simulink model "simulacao"  (R2020b)
settings: Solver=VariableStepAuto  StartTime=0.0  StopTime=10.0  RelTol=1e-3
values from neighbouring files (symbols this model uses):
  i = 1    [teste.m]    (also in teste2.m)
  ki0 = 0.1    [teste.m]    (also in teste2.m = 0.2)
  kp0 = 0.1    [teste.m]    (also in teste2.m = 0.5)
  T = 0.01    [teste.m]    (also in teste2.m)
libraries: simulink x1
settings Model: Creator=luanh  LastModifiedBy=luanaraujo
settings DebuggingCC: AlgebraicLoopMsg=none

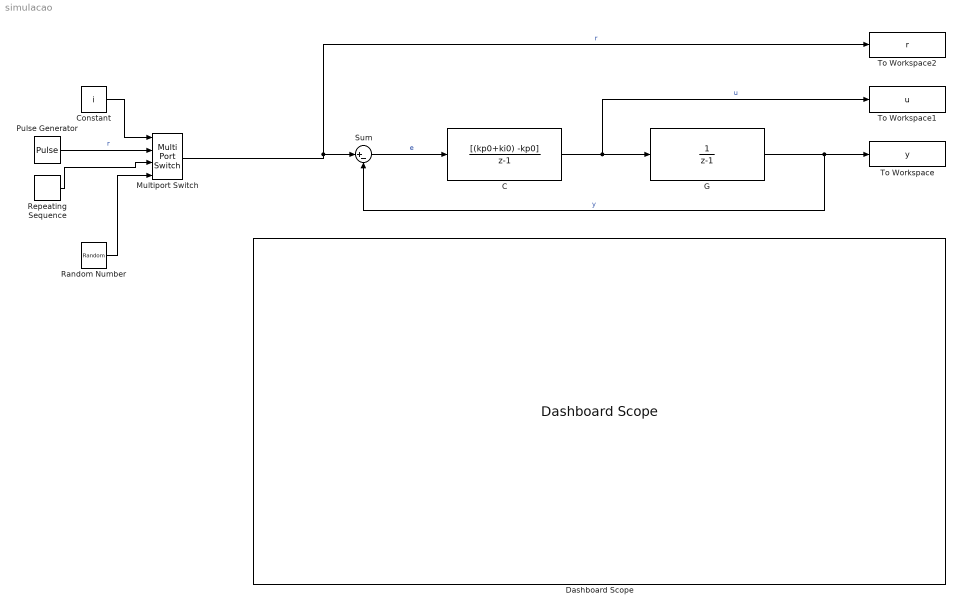
== system simulacao ==
  C : DiscreteTransferFcn  Numerator=[(kp0+ki0) -kp0]  Denominator=[1 -1]  SampleTime=T
  Constant : Constant  Value=i
  Dashboard Scope : DashboardScope
  G : DiscreteTransferFcn  Denominator=[1 -1]  SampleTime=T
  Multiport Switch : MultiPortSwitch
  Pulse Generator : DiscretePulseGenerator  PulseType=Time based  PulseWidth=50
  Random Number : RandomNumber  SampleTime=1
  Repeating Sequence : simulink/Sources/Repeating Sequence  rep_seq_t=[0 2]  rep_seq_y=[0 2]
  Sum : Sum  Inputs=|+-
  To Workspace : ToWorkspace  VariableName=y  SaveFormat=Timeseries  SampleTime=T
  To Workspace1 : ToWorkspace  VariableName=u  SaveFormat=Timeseries  SampleTime=T
  To Workspace2 : ToWorkspace  VariableName=r  SaveFormat=Timeseries  SampleTime=T
  wires:
  Sum/1 -> C/1  "e"
  C/1 -> To Workspace1/1, G/1  "u"
  G/1 -> To Workspace/1, Sum/2  "y"
  Multiport Switch/1 -> To Workspace2/1, Sum/1  "r"
  Pulse Generator/1 -> Multiport Switch/2  "r"
  Constant/1 -> Multiport Switch/1
  Repeating Sequence/1 -> Multiport Switch/3
  Random Number/1 -> Multiport Switch/4
